simulink model "wheel"  (R2018b)
settings: Solver=VariableStepAuto  StartTime=0.0  StopTime=10.0  RelTol=1e-3
values from neighbouring files (symbols this model uses):
  J_w = 0.01    [dane.m]    (also in untitled.m)
  r_w = 0.3    [dane.m]    (also in untitled.m)
  v0 = 28    [dane.m]
settings Model: Creator=lpa1  LastModifiedBy=lpa1

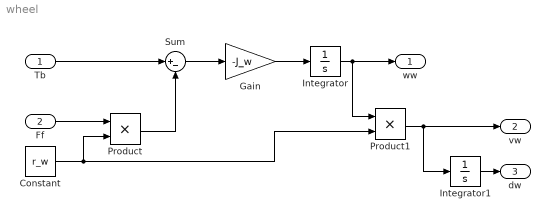
== system wheel ==
  "Tb " : Inport
  "Ff " : Inport  Port=2
  Constant : Constant  Value=r_w
  Gain : Gain  Gain=-J_w
  Integrator : Integrator  InitialCondition=v0/r_w  LimitOutput=on  UpperSaturationLimit=1000  LowerSaturationLimit=0
  Integrator1 : Integrator
  Product : Product
  Product1 : Product
  Sum : Sum  Inputs=|+-
  ww : Outport
  "vw " : Outport  Port=2
  "dw " : Outport  Port=3
  wires:
  "Tb "/1 -> Sum/1
  "Ff "/1 -> Product/1
  Constant/1 -> Product1/2, Product/2
  Product/1 -> Sum/2
  Sum/1 -> Gain/1
  Gain/1 -> Integrator/1
  Integrator/1 -> Product1/1, ww/1
  Product1/1 -> Integrator1/1, "vw "/1
  Integrator1/1 -> "dw "/1
